simulink model "temp_control"  (R2018a)
settings: Solver=VariableStepAuto  StartTime=0.0  StopTime=10.0  RelTol=1e-3
settings Model: Creator=arturogilaparicio  LastModifiedBy=arturogilaparicio

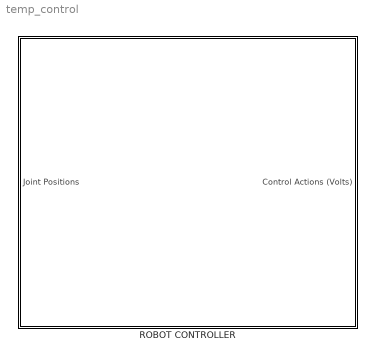
== system temp_control ==
  ROBOT CONTROLLER : Subsystem  Description=ROBOT CONTROLLER
      mask Display:
      | port_label('output', 1, 'Control Actions')
      | port_label('input', 1, 'Joint Positions')
      | image(imread('images/robot-controller.jpg'))

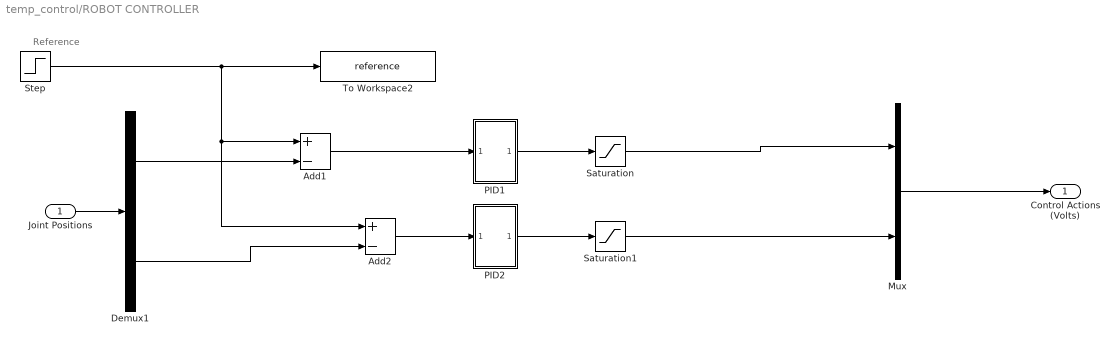
== system temp_control/ROBOT CONTROLLER ==
  note: Reference
  Joint Positions : Inport  PortDimensions=6
  Add1 : Sum  Inputs=+-
  Add2 : Sum  Inputs=+-
  Demux1 : Demux  Outputs=2
  Mux : Mux  Inputs=2
  PID1 : Subsystem
  "PID2 " : Subsystem
  Saturation : Saturate  UpperLimit=48  LowerLimit=-48
  Saturation1 : Saturate  UpperLimit=48  LowerLimit=-48
  Step : Step  Time=0  After=0.3  SampleTime=0
  To Workspace2 : ToWorkspace  VariableName=reference  SampleTime=-1
  Control Actions (Volts) : Outport
  wires:
  Saturation1/1 -> Mux/2
  Saturation/1 -> Mux/1
  Add2/1 -> "PID2 "/1(In1)
  Step/1 -> To Workspace2/1, Add1/1, Add2/1
  Joint Positions/1 -> Demux1/1
  Demux1/1 -> Add1/2
  Demux1/2 -> Add2/2
  Mux/1 -> Control Actions (Volts)/1
  PID1/1(Out1) -> Saturation/1
  Add1/1 -> PID1/1(In1)
  "PID2 "/1(Out1) -> Saturation1/1

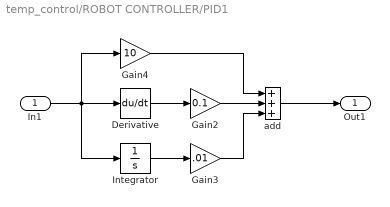
== system temp_control/ROBOT CONTROLLER/PID1 ==
  In1 : Inport
  Derivative : Derivative
  Gain2 : Gain  Gain=0.1
  Gain3 : Gain  Gain=.01
  Gain4 : Gain  Gain=10
  Integrator : Integrator
  add : Sum  Inputs=+++
  Out1 : Outport
  wires:
  add/1 -> Out1/1
  Gain4/1 -> add/1
  Gain2/1 -> add/2
  Derivative/1 -> Gain2/1
  Gain3/1 -> add/3
  Integrator/1 -> Gain3/1
  In1/1 -> Integrator/1, Gain4/1, Derivative/1

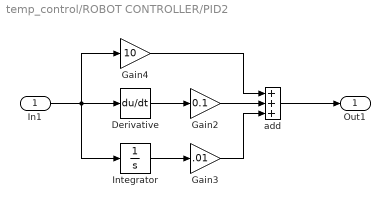
== system temp_control/ROBOT CONTROLLER/PID2  ==
  In1 : Inport
  Derivative : Derivative
  Gain2 : Gain  Gain=0.1
  Gain3 : Gain  Gain=.01
  Gain4 : Gain  Gain=10
  Integrator : Integrator
  add : Sum  Inputs=+++
  Out1 : Outport
  wires:
  add/1 -> Out1/1
  Gain4/1 -> add/1
  Gain2/1 -> add/2
  Derivative/1 -> Gain2/1
  Gain3/1 -> add/3
  Integrator/1 -> Gain3/1
  In1/1 -> Integrator/1, Gain4/1, Derivative/1
